simulink model "actividad2"  (R2021a)
settings: Solver=VariableStepAuto  StartTime=0.0  StopTime=30.0  RelTol=1e-3
settings Model: Creator=Agus  LastModifiedBy=valen

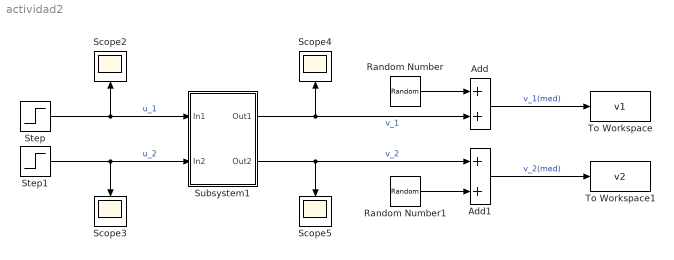
== system actividad2 ==
  Add : Sum
  Add1 : Sum
  Random Number : RandomNumber  Variance=1e-6  SampleTime=0.1
  Random Number1 : RandomNumber  Variance=1e-6  SampleTime=0.1
  Scope{2..5} (4 alike) : Scope
  Step : Step  After=0  SampleTime=0
  Step1 : Step  After=0  SampleTime=0
  Subsystem1 : Subsystem  mask{a1=0.15, a2=0.2, b1=0.3, b2=0.5, c1=0.3, c2=-0.4, d1=6, d2=20}
  To Workspace : ToWorkspace  VariableName=v1  SaveFormat=Timeseries  SampleTime=-1
  To Workspace1 : ToWorkspace  VariableName=v2  SaveFormat=Timeseries  SampleTime=-1
  wires:
  Step/1 -> Scope2/1, Subsystem1/1(In1)  "u_1"
  Step1/1 -> Scope3/1, Subsystem1/2(In2)  "u_2"
  Subsystem1/1(Out1) -> Add/2, Scope4/1  "v_1"
  Subsystem1/2(Out2) -> Add1/1, Scope5/1  "v_2"
  Add1/1 -> To Workspace1/1  "v_2(med)"
  Add/1 -> To Workspace/1  "v_1(med)"
  Random Number1/1 -> Add1/2
  Random Number/1 -> Add/1

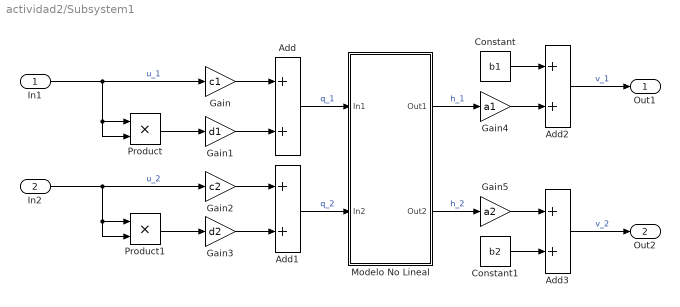
== system actividad2/Subsystem1 ==
  In1 : Inport
  In2 : Inport  Port=2
  Add{,1..3} (4 alike) : Sum
  Constant : Constant  Value=b1
  Constant1 : Constant  Value=b2
  Gain : Gain  Gain=c1
  Gain1 : Gain  Gain=d1
  Gain2 : Gain  Gain=c2
  Gain3 : Gain  Gain=d2
  Gain4 : Gain  Gain=a1
  Gain5 : Gain  Gain=a2
  Modelo No Lineal : Subsystem  mask{A=100, K=15, h10=20, h20=10}
      mask prompts: A "Area"; h10 "Altura Inicial 1"; h20 "Altura Inicial 2"
  Product : Product
  Product1 : Product
  Out1 : Outport
  Out2 : Outport  Port=2
  wires:
  Add3/1 -> Out2/1  "v_2"
  Modelo No Lineal/1(Out1) -> Gain4/1  "h_1"
  In2/1 -> Product1/1, Product1/2, Gain2/1  "u_2"
  Constant/1 -> Add2/1
  Gain5/1 -> Add3/1
  Gain3/1 -> Add1/2
  Constant1/1 -> Add3/2
  In1/1 -> Product/2, Product/1, Gain/1  "u_1"
  Gain/1 -> Add/1
  Modelo No Lineal/2(Out2) -> Gain5/1  "h_2"
  Product1/1 -> Gain3/1
  Gain2/1 -> Add1/1
  Add1/1 -> Modelo No Lineal/2(In2)  "q_2"
  Add2/1 -> Out1/1  "v_1"
  Product/1 -> Gain1/1
  Gain4/1 -> Add2/2
  Gain1/1 -> Add/2
  Add/1 -> Modelo No Lineal/1(In1)  "q_1"

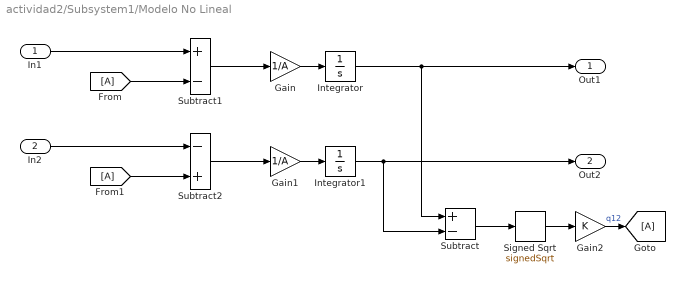
== system actividad2/Subsystem1/Modelo No Lineal ==
  In1 : Inport
  In2 : Inport  Port=2
  Gain : Gain  Gain=1/A
  Gain1 : Gain  Gain=1/A
  Gain2 : Gain  Gain=K
  Integrator : Integrator  InitialCondition=h10
  Integrator1 : Integrator  InitialCondition=h20
  Signed Sqrt : Sqrt  Operator=signedSqrt  SaturateOnIntegerOverflow=on
  Subtract : Sum  Inputs=+-
  Subtract1 : Sum  Inputs=+-
  Subtract2 : Sum  Inputs=-+
  Out1 : Outport
  Out2 : Outport  Port=2
  wires:
  In2/1 -> Subtract2/1
  [A] -> Subtract2/2
  Gain/1 -> Integrator/1
  [A] -> Subtract1/2
  Subtract/1 -> Signed Sqrt/1
  Integrator/1 -> Out1/1, Subtract/1
  Signed Sqrt/1 -> Gain2/1
  Integrator1/1 -> Out2/1, Subtract/2
  Subtract2/1 -> Gain1/1
  Gain2/1 -> [A]  "q12"
  In1/1 -> Subtract1/1
  Gain1/1 -> Integrator1/1
  Subtract1/1 -> Gain/1
